simulink model "tri4"  (R2016b)
settings: Solver=VariableStepAuto  StartTime=0.0  StopTime=20  RelTol=1e-3
settings Model: Creator=Admin  LastModifiedBy=Admin

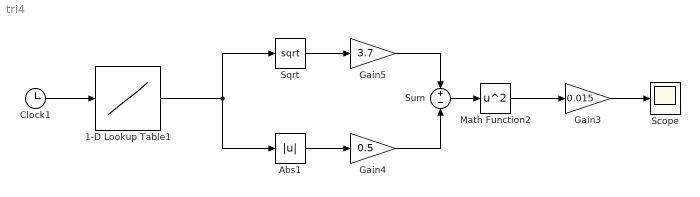
== system tri4 ==
  1-D Lookup Table1 : Lookup_n-D  NumberOfTableDimensions=1  BreakpointsForDimension1=[0,1.15,2.3,4.17,19.3,24.5]  Table=[0,1.3,3.1,6.2,11.15,25]  InternalRulePriority=Speed  RndMeth=Simplest  InputSameDT=on
  Abs1 : Abs
  Clock1 : Clock
  Gain3 : Gain  Gain=0.015
  Gain4 : Gain  Gain=0.5
  Gain5 : Gain  Gain=3.7
  Math Function2 : Math  Operator=square  SaturateOnIntegerOverflow=on
  Scope : Scope
  Sqrt : Sqrt  SaturateOnIntegerOverflow=on
  Sum : Sum  Inputs=+|-
  wires:
  Clock1/1 -> 1-D Lookup Table1/1
  1-D Lookup Table1/1 -> Sqrt/1, Abs1/1
  Math Function2/1 -> Gain3/1
  Gain3/1 -> Scope/1
  Sum/1 -> Math Function2/1
  Gain5/1 -> Sum/1
  Gain4/1 -> Sum/2
  Abs1/1 -> Gain4/1
  Sqrt/1 -> Gain5/1
